simulink model "aocs"  (R2026a)
settings: Solver=VariableStepAuto  StopTime=200
values from neighbouring files (symbols this model uses):
  A = [0, 0, 0, 1, 0, 0 ... (first row only)    [aocs_controller.m]    (also in attempt999999.m; untitled.m = [0,0,0,1,0,0)
  B = [zeros(3,3) ... (first row only)    [aocs_controller.m]    (also in attempt999999.m; untitled.m = [zeros(3,3); inv(I)])
  C = eye(6, 6)    [aocs_controller.m]    (also in attempt999999.m = eye(6); untitled.m = eye(6))
  D = zeros(6, 3)    [aocs_controller.m]    (also in attempt999999.m = zeros(6,3); untitled.m = zeros(6,3))
  K = lqr(A,B,Q,R_c)    [aocs_controller.m]
  Ki = K_aug(:, na+1:end)    [attempt999999.m]    (also in untitled.m)
  Kx = K_aug(:,1:n)    [aocs_controller.m]    (also in attempt999999.m = K_aug(:, 1:na); untitled.m = K_aug(:, 1:na))
  omega_0 = 7.272 * 10^-5    (= 7.272e-05)    [attempt999999.m]
settings Model: Creator=syane  LastModifiedBy=syane

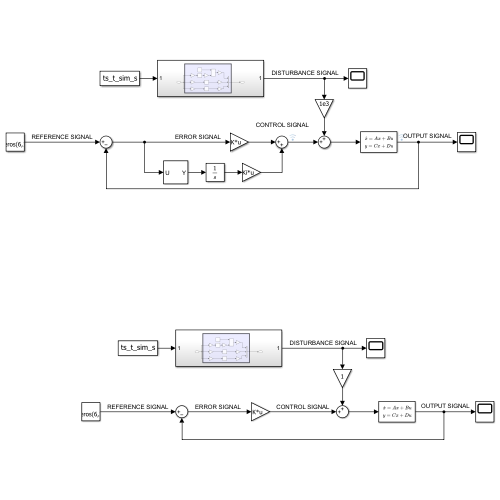
[thumbnail: Simulink's stored preview of the top-level diagram]
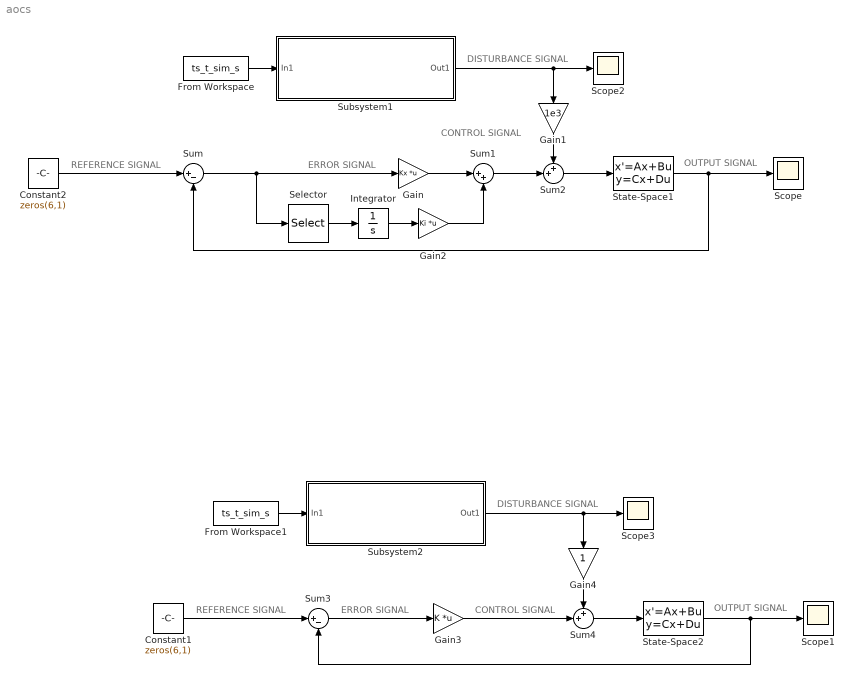
== system aocs ==
  note: DISTURBANCE SIGNAL
  note: CONTROL SIGNAL
  note: ERROR SIGNAL
  note: OUTPUT SIGNAL
  note: REFERENCE SIGNAL
  note: REFERENCE SIGNAL
  note: ERROR SIGNAL
  note: OUTPUT SIGNAL
  note: DISTURBANCE SIGNAL
  note: CONTROL SIGNAL
  Constant1 : Constant  Value=zeros(6,1)
  Constant2 : Constant  Value=zeros(6,1)
  From Workspace : FromWorkspace  VariableName=ts_t_sim_s
  From Workspace1 : FromWorkspace  VariableName=ts_t_sim_s
  Gain : Gain  Gain=Kx  Multiplication=Matrix(K*u)
  Gain1 : Gain  Gain=1e3
  Gain2 : Gain  Gain=Ki  Multiplication=Matrix(K*u)
  Gain3 : Gain  Gain=K  Multiplication=Matrix(K*u)
  Gain4 : Gain
  Integrator : Integrator  InitialCondition=zeros(3,1)
  Scope{,1..3} (4 alike) : Scope
      Scope settings: ActiveDisplayYMinimum=-1.271014252230675E+13  ActiveDisplayYMaximum=1.1439128215125742E+14
      Scope1 settings: ActiveDisplayYMinimum=-7.1748704481466792E-5  ActiveDisplayYMaximum=0.00012380945389570797  YLabel=Kinematic State
      Scope2 settings: ActiveDisplayYMinimum=1.9082709998725175E-5  ActiveDisplayYMaximum=2.1622646412244377E-5  DataLoggingVariableName=ScopeData2
      Scope3 settings: ActiveDisplayYMinimum=1.9082709998725175E-5  ActiveDisplayYMaximum=2.1622646412244377E-5  DataLoggingVariableName=ScopeData3
  Selector : Selector  InputPortWidth=6  IndexOptions=Index vector (dialog)  Indices=[1 2 3]  OutputSizes=1
  State-Space1 : StateSpace  A=A  B=B  C=C  D=D  InitialCondition=0
  State-Space2 : StateSpace  A=A  B=B  C=C  D=D  InitialCondition=0
  Subsystem1 : Subsystem
  Subsystem2 : Subsystem
  Sum : Sum  Inputs=|+-
  Sum1 : Sum  Inputs=|++
  Sum2 : Sum  Inputs=++|
  Sum3 : Sum  Inputs=|+-
  Sum4 : Sum  Inputs=++|
  wires:
  State-Space1/1 -> Scope/1, Sum/2
  Constant2/1 -> Sum/1
  Sum2/1 -> State-Space1/1
  From Workspace/1 -> Subsystem1/1(In1)
  Subsystem1/1(Out1) -> Scope2/1, Gain1/1
  Gain1/1 -> Sum2/1
  Sum/1 -> Gain/1, Selector/1
  Gain4/1 -> Sum4/1
  Subsystem2/1(Out1) -> Scope3/1, Gain4/1
  From Workspace1/1 -> Subsystem2/1(In1)
  Gain3/1 -> Sum4/2
  Sum4/1 -> State-Space2/1
  Sum3/1 -> Gain3/1
  Constant1/1 -> Sum3/1
  State-Space2/1 -> Scope1/1, Sum3/2
  Integrator/1 -> Gain2/1
  Sum1/1 -> Sum2/2
  Gain/1 -> Sum1/1
  Gain2/1 -> Sum1/2
  Selector/1 -> Integrator/1

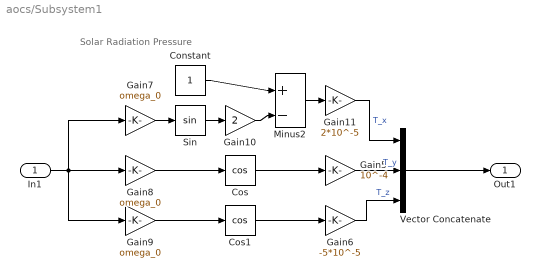
== system aocs/Subsystem1 ==
  note: Solar Radiation Pressure
  In1 : Inport
  Constant : Constant
  Cos : Trigonometry  Operator=cos
  Cos1 : Trigonometry  Operator=cos
  Gain10 : Gain  Gain=2
  Gain11 : Gain  Gain=2*10^-5
  Gain5 : Gain  Gain=10^-4
  Gain6 : Gain  Gain=-5*10^-5
  Gain7 : Gain  Gain=omega_0
  Gain8 : Gain  Gain=omega_0
  Gain9 : Gain  Gain=omega_0
  Minus2 : Sum  Inputs=+|-
  Sin : Trigonometry
  Vector Concatenate : Concatenate  NumInputs=3
  Out1 : Outport
  wires:
  In1/1 -> Gain7/1, Gain9/1, Gain8/1
  Sin/1 -> Gain10/1
  Gain10/1 -> Minus2/2
  Gain7/1 -> Sin/1
  Cos/1 -> Gain5/1
  Vector Concatenate/1 -> Out1/1
  Minus2/1 -> Gain11/1
  Gain8/1 -> Cos/1
  Gain5/1 -> Vector Concatenate/2  "T_y"
  Gain6/1 -> Vector Concatenate/3  "T_z"
  Cos1/1 -> Gain6/1
  Gain9/1 -> Cos1/1
  Constant/1 -> Minus2/1
  Gain11/1 -> Vector Concatenate/1  "T_x"

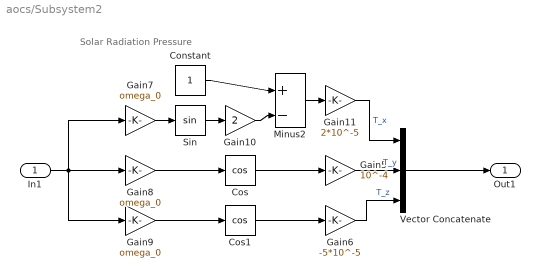
== system aocs/Subsystem2 ==
  note: Solar Radiation Pressure
  In1 : Inport
  Constant : Constant
  Cos : Trigonometry  Operator=cos
  Cos1 : Trigonometry  Operator=cos
  Gain10 : Gain  Gain=2
  Gain11 : Gain  Gain=2*10^-5
  Gain5 : Gain  Gain=10^-4
  Gain6 : Gain  Gain=-5*10^-5
  Gain7 : Gain  Gain=omega_0
  Gain8 : Gain  Gain=omega_0
  Gain9 : Gain  Gain=omega_0
  Minus2 : Sum  Inputs=+|-
  Sin : Trigonometry
  Vector Concatenate : Concatenate  NumInputs=3
  Out1 : Outport
  wires:
  In1/1 -> Gain7/1, Gain9/1, Gain8/1
  Sin/1 -> Gain10/1
  Gain10/1 -> Minus2/2
  Gain7/1 -> Sin/1
  Cos/1 -> Gain5/1
  Vector Concatenate/1 -> Out1/1
  Minus2/1 -> Gain11/1
  Gain8/1 -> Cos/1
  Gain5/1 -> Vector Concatenate/2  "T_y"
  Gain6/1 -> Vector Concatenate/3  "T_z"
  Cos1/1 -> Gain6/1
  Gain9/1 -> Cos1/1
  Constant/1 -> Minus2/1
  Gain11/1 -> Vector Concatenate/1  "T_x"
